simulink model "bolide_modele_simul3_p"  (R2023b)
settings: Solver=VariableStepAuto  StartTime=0.0  StopTime=20  RelTol=1e-3
model workspace (MATLAB code in the model file):
  | %% True Parameters
  | % Masses
  | mw=0.1;
  | mb=1;
  | M=1.2;
  | 
  | % Distances
  | rho=0.07;
  | l=0.02;
  | d=0.015; % distance A-C
  | 
  | % Electriques
  | L=0.05;
  | R=1e6;
  | % r;
  | 
  | % Couples
  | k=2.63e4;
  | % alpha=34.6;
  | % beta=2.06e5;
  | 
  | % Moments inertie
  | Iwy=2.45e-4;
  | Ipsi=1.53e-2;
  | 
  | % Utilitaire
  | beta = (M + 2*Iwy/rho^2);
  | gamma = Ipsi + mb*d^2;
  | 
  | %% Nominal Equilibrium Trajectory
  | 
  | 
  | 
  | Ubar = 12;
  | Urbar = Ubar;
  | Ulbar = Ubar;
  | 
  | ubar = rho/2/k*Ubar; % m/s
  | psibar = 0;
  | vbar = 0;
  | irbar = 0;
  | ilbar = 0;
  | 
  | statebar = [0; ubar; psibar; vbar; irbar; ilbar];
  | 
  | % function res = p(t)
  | %     res = ubar*t;
  | % end
  | 
  | % function res = statebar(t)
  | %    statebar = [p(t); ubar; psibar; vbar; irbar; ilbar];
  | % end
settings Model: Creator=Jules  LastModifiedBy=Jules

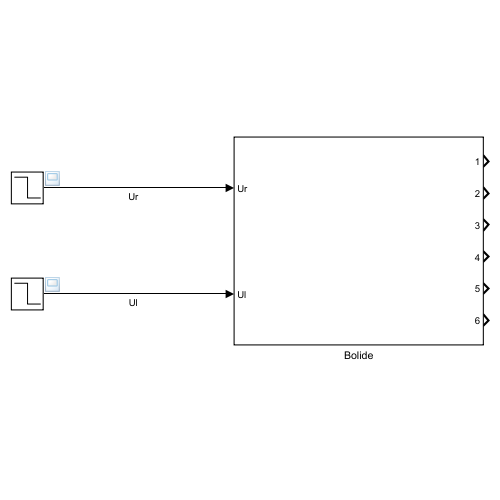
[thumbnail: Simulink's stored preview of the top-level diagram]
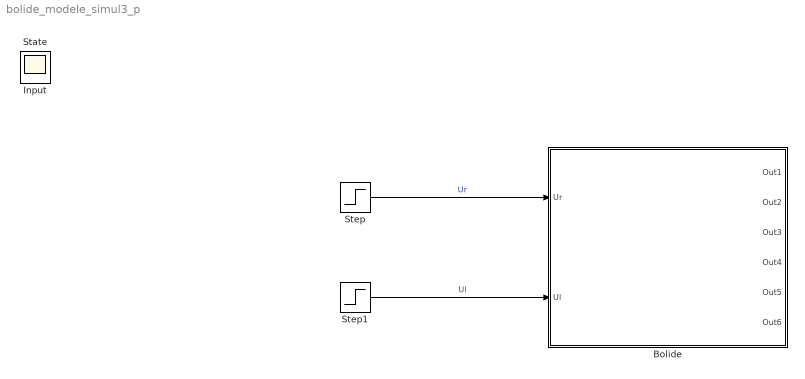
== system bolide_modele_simul3_p ==
  Bolide : Subsystem
  Step : Step  Before=Urbar  After=Urbar - 0.1  SampleTime=0
  Step1 : Step  Time=3  Before=Ulbar  After=Ulbar - 0.3  SampleTime=0
  Input : Scope
  State : Scope
  wires:
  Step/1 -> Bolide/1(Ur)  "Ur"
  Step1/1 -> Bolide/2(Ul)  "Ul"

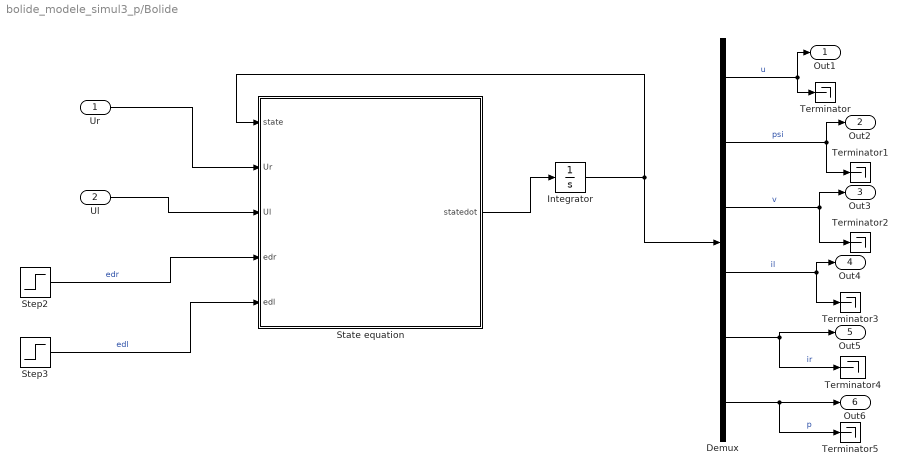
== system bolide_modele_simul3_p/Bolide ==
  Ur : Inport
  Ul : Inport  Port=2
  Demux : Demux  Outputs=6
  Integrator : Integrator  InitialCondition=statebar
  State equation : MATLAB Function  TreatAsAtomicUnit=on
  Step2 : Step  After=0  SampleTime=0
  Step3 : Step  After=0  SampleTime=0
  Terminator{,1..5} (6 alike) : Terminator
  Out1 : Outport
  Out2 : Outport  Port=2
  Out3 : Outport  Port=3
  Out4 : Outport  Port=4
  Out5 : Outport  Port=5
  Out6 : Outport  Port=6
  wires:
  Step3/1 -> State equation/5(edl)  "edl"
  State equation/1(statedot) -> Integrator/1
  Integrator/1 -> State equation/1(state), Demux/1
  Demux/1 -> Terminator/1, Out1/1  "u"
  Demux/4 -> Out4/1, Terminator3/1  "il"
  Demux/5 -> Terminator4/1, Out5/1  "ir"
  Demux/2 -> Out2/1, Terminator1/1  "psi"
  Demux/3 -> Terminator2/1, Out3/1  "v"
  Step2/1 -> State equation/4(edr)  "edr"
  Ul/1 -> State equation/3(Ul)
  Ur/1 -> State equation/2(Ur)
  Demux/6 -> Out6/1, Terminator5/1  "p"

== matlab function bolide_modele_simul3_p/Bolide/State equation ==
  data: state input; statedot output; Ur input; Ul input; edr input; edl input; M parameter; rho parameter; l parameter; Iwy parameter; Ipsi parameter; d parameter; L parameter; R parameter; k parameter; mb parameter; beta parameter; gamma parameter
function statedot = fcn(state,Ur, Ul, edr, edl, M, rho, l, Iwy, Ipsi, d, L, R, k, mb, beta, gamma)
% ed est l'entrée de perturbation, != d (distance AC)
% Model parameters M,Ipsi,d,L,R,k defined in "Model Explorer/Matlab Code"

p = state(1); % intégrale temporelle de u, distance parcourue
u = state(2);
psi = state(3);
v = state(4); % psidot
ir = state(5); % Intensité à gauche
il = state(6);

is = ir + il; % Somme
id = ir - il; % Diff
Us = Ur + Ul + edr + edl;
Ud = Ur - Ul + edr - edl;

pdot = u
udot = 1/beta*(k/rho*is - mb*d*v^2);
psidot = v;
vdot = 1/gamma*(l*k/(2*rho)*id + mb*d*u*v);
isdot = 1/L*(Us - R*is - 2*k/rho*u);
iddot = 1/L*(Ud - R*id - k*l/rho*v);

irdot = 0.5*(isdot + iddot);
ildot = 0.5*(isdot - iddot);

statedot = [pdot; udot; psidot; vdot; irdot; ildot];
